simulink library "HDL_ieee_8021513"  (R2024a)
settings: Solver=FixedStepDiscrete  StartTime=0.0  StopTime=10.0  RelTol=1e-3
undefined symbols (not defined in the file): Add, axiWidth, CONST, fs, peakDetectorThreshold, peakDetectorWindow, QAM, Shift
libraries: hdlsllib x199, $bdroot x91, whdlutilities x34, whdledac x9, simulink x8, whdlmod x6, dspsigops x5, dsphdlfiltering2 x4, embreciprocals x3, dsphdlsigops2 x2, commhdlcrc x2, dspstat3 x2
(part 6 of 6)

== system HDL_ieee_8021513/full_tx/store_frame_in_ram/read_frame_from_ram/bits_selector ==
  rd_addr : Inport
  bits_per_subcarrier : Inport  Port=2
  Compare To Constant : hdlsllib/Logic and Bit Operations/Compare To Constant  relop=<=  const=CONST.preambleDataCarriers-1  OutDataTypeStr=boolean
  Compare To Constant1 : hdlsllib/Logic and Bit Operations/Compare To Constant  relop=<=  const=CONST.preambleDataCarriers + CONST.channelDataCarriers -1  OutDataTypeStr=boolean
  Compare To Constant2 : hdlsllib/Logic and Bit Operations/Compare To Constant  relop=<=  const=CONST.preambleDataCarriers + CONST.channelDataCarriers + CONST.headerDataCarriers-1  OutDataTypeStr=boolean
  Constant : Constant  OutDataTypeStr=fixdt(0,4,0)  SampleTime=-1
  Constant1 : Constant  OutDataTypeStr=fixdt(0,4,0)  SampleTime=-1
  Constant2 : Constant  Value=2  OutDataTypeStr=fixdt(0,4,0)  SampleTime=-1
  Delay{,1..5} (6 alike) : Delay  DelayLength=1  InitialCondition=0  UseCircularBuffer=on
  Multiport Switch : MultiPortSwitch  DataPortOrder=Zero-based contiguous  Inputs=4  zeroidx=on  SaturateOnIntegerOverflow=off  InputSameDT=off
  State Control : StateControl  StateControl=Synchronous
  one_hot_coder : Subsystem
  bits_per_subcarrier_out : Outport
  wires:
  Delay5/1 -> one_hot_coder/1(preamble)
  Delay4/1 -> one_hot_coder/2(channel)
  Delay3/1 -> one_hot_coder/3(header)
  Delay2/1 -> Delay1/1
  Delay1/1 -> Multiport Switch/5
  Compare To Constant1/1 -> Delay4/1
  one_hot_coder/1(bits_per_subcarrier_select) -> Delay/1
  Compare To Constant/1 -> Delay5/1
  Constant2/1 -> Multiport Switch/4
  Constant1/1 -> Multiport Switch/3
  Constant/1 -> Multiport Switch/2
  Compare To Constant2/1 -> Delay3/1
  rd_addr/1 -> Compare To Constant2/1, Compare To Constant/1, Compare To Constant1/1
  Multiport Switch/1 -> bits_per_subcarrier_out/1
  Delay/1 -> Multiport Switch/1
  bits_per_subcarrier/1 -> Delay2/1

== system HDL_ieee_8021513/full_tx/store_frame_in_ram/read_frame_from_ram/cp_len_creator ==
  rd_addr : Inport
  cp_len_in : Inport  Port=2
  Bits to Word : hdlsllib/Logic and Bit Operations/Bits to Word
  Compare To Constant : hdlsllib/Logic and Bit Operations/Compare To Constant  relop=<=  const=CONST.preambleDataCarriers-1  OutDataTypeStr=boolean
  Compare To Constant1 : hdlsllib/Logic and Bit Operations/Compare To Constant  relop=<=  const=CONST.preambleDataCarriers + CONST.channelDataCarriers -1  OutDataTypeStr=boolean
  Compare To Constant2 : hdlsllib/Logic and Bit Operations/Compare To Constant  relop=<=  const=CONST.preambleDataCarriers + CONST.channelDataCarriers + CONST.headerDataCarriers-1  OutDataTypeStr=boolean
  Constant : Constant  Value=CONST.preambleCyclicPrefixLen  OutDataTypeStr=uint8  SampleTime=-1
  Constant1 : Constant  Value=CONST.channelCyclicPrefixLen  OutDataTypeStr=uint8  SampleTime=-1
  Constant2 : Constant  Value=CONST.headerCyclicPrefixLen  OutDataTypeStr=uint8  SampleTime=-1
  Constant3 : Constant  Value=CONST.N/32  OutDataTypeStr=fixdt(0,4,0)  SampleTime=-1
  Data Type Conversion : DataTypeConversion  OutDataTypeStr=fixdt(0,1,0)  SaturateOnIntegerOverflow=off  RndMeth=Floor
  Delay{,1..5} (6 alike) : Delay  DelayLength=1  InitialCondition=0  UseCircularBuffer=on
  Delay6 : Delay  InitialCondition=0  UseCircularBuffer=on
  Multiport Switch : MultiPortSwitch  DataPortOrder=Zero-based contiguous  Inputs=4  zeroidx=on  OutDataTypeStr=uint8  SaturateOnIntegerOverflow=off
  Product : Product  OutDataTypeStr=uint8
  State Control : StateControl  StateControl=Synchronous
  one_hot_coder : Subsystem
  cp_len : Outport
  wires:
  Delay6/1 -> Product/2
  Delay5/1 -> one_hot_coder/1(preamble)
  Delay4/1 -> one_hot_coder/2(channel)
  Delay3/1 -> one_hot_coder/3(header)
  Delay2/1 -> Delay1/1
  rd_addr/1 -> Compare To Constant2/1, Compare To Constant/1, Compare To Constant1/1
  Compare To Constant/1 -> Delay5/1
  Compare To Constant1/1 -> Delay4/1
  Compare To Constant2/1 -> Delay3/1
  Constant/1 -> Multiport Switch/2
  Constant1/1 -> Multiport Switch/3
  Constant2/1 -> Multiport Switch/4
  Multiport Switch/1 -> cp_len/1
  one_hot_coder/1(cp_select) -> Delay/1
  Delay/1 -> Multiport Switch/1
  Constant3/1 -> Product/1
  cp_len_in/1 -> Data Type Conversion/1
  Product/1 -> Delay2/1
  Data Type Conversion/1 -> Bits to Word/1
  Bits to Word/1 -> Delay6/1
  Delay1/1 -> Multiport Switch/5

== system HDL_ieee_8021513/full_tx/store_frame_in_ram/read_frame_from_ram/init_selector ==
  rd_addr : Inport
  Compare To Constant : hdlsllib/Logic and Bit Operations/Compare To Constant  relop=<=  const=CONST.preambleDataCarriers-1  OutDataTypeStr=boolean
  Compare To Constant1 : hdlsllib/Logic and Bit Operations/Compare To Constant  relop=<=  const=CONST.preambleDataCarriers + CONST.channelDataCarriers -1  OutDataTypeStr=boolean
  Compare To Constant2 : hdlsllib/Logic and Bit Operations/Compare To Constant  relop=<=  const=CONST.preambleDataCarriers + CONST.channelDataCarriers + CONST.headerDataCarriers-1  OutDataTypeStr=boolean
  Constant : Constant  Value=CONST.preambleScramblerInit  OutDataTypeStr=boolean  SampleTime=-1
  Constant1 : Constant  Value=CONST.channelScramblerInit  OutDataTypeStr=boolean  SampleTime=-1
  Constant2 : Constant  Value=CONST.headerScramblerInit  OutDataTypeStr=boolean  SampleTime=-1
  Constant3 : Constant  Value=CONST.payloadScramblerInit  OutDataTypeStr=boolean  SampleTime=-1
  Delay{,1..3} (4 alike) : Delay  DelayLength=1  InitialCondition=0  UseCircularBuffer=on
  Multiport Switch : MultiPortSwitch  DataPortOrder=Zero-based contiguous  Inputs=4  zeroidx=on  SaturateOnIntegerOverflow=off  InputSameDT=off
  State Control : StateControl  StateControl=Synchronous
  one_hot_coder : Subsystem
  init : Outport
  wires:
  Delay3/1 -> one_hot_coder/1(preamble)
  Delay2/1 -> one_hot_coder/2(channel)
  Delay1/1 -> one_hot_coder/3(header)
  Compare To Constant1/1 -> Delay2/1
  one_hot_coder/1(cp_select) -> Delay/1
  Compare To Constant/1 -> Delay3/1
  Constant2/1 -> Multiport Switch/4
  Constant1/1 -> Multiport Switch/3
  Constant/1 -> Multiport Switch/2
  Compare To Constant2/1 -> Delay1/1
  rd_addr/1 -> Compare To Constant2/1, Compare To Constant/1, Compare To Constant1/1
  Multiport Switch/1 -> init/1
  Delay/1 -> Multiport Switch/1
  Constant3/1 -> Multiport Switch/5

== system HDL_ieee_8021513/full_tx/store_frame_in_ram/write_frame_to_ram/ram_formatting ==
  preamble_valid : Inport
  channel_valid : Inport  Port=2
  header_valid : Inport  Port=3
  payload_valid : Inport  Port=4
  preamble : Inport  Port=5
  channel : Inport  Port=6
  header : Inport  Port=7
  payload : Inport  Port=8
  Bit Concat{,1..2,6} (4 alike) : hdlsllib/Logic and Bit Operations/Bit Concat  numInputs=2
  Constant10 : Constant  Value=0  OutDataTypeStr=boolean  SampleTime=-1
  Constant11 : Constant  Value=0  OutDataTypeStr=boolean  SampleTime=-1
  Demux : Demux  Outputs=2
  Demux3 : Demux  Outputs=2
  Multiport Switch : MultiPortSwitch  DataPortOrder=Zero-based contiguous  Inputs=4  zeroidx=on  SaturateOnIntegerOverflow=off  InputSameDT=off
  State Control : StateControl  StateControl=Synchronous
  one_hot_coder : Subsystem
  Out1 : Outport
  wires:
  Demux3/2 -> Bit Concat6/2
  Demux3/1 -> Bit Concat6/1
  Demux/2 -> Bit Concat2/2
  Demux/1 -> Bit Concat2/1
  channel/1 -> Bit Concat1/2
  Constant11/1 -> Bit Concat1/1
  preamble/1 -> Bit Concat/2
  Constant10/1 -> Bit Concat/1
  header_valid/1 -> one_hot_coder/3(header_valid)
  Bit Concat1/1 -> Multiport Switch/3
  Bit Concat2/1 -> Multiport Switch/4
  header/1 -> Demux/1
  payload/1 -> Demux3/1
  one_hot_coder/1(data_select) -> Multiport Switch/1  "data_select"
  Bit Concat6/1 -> Multiport Switch/5
  channel_valid/1 -> one_hot_coder/2(channel_valid)
  preamble_valid/1 -> one_hot_coder/1(preamble_valid)
  Multiport Switch/1 -> Out1/1
  payload_valid/1 -> one_hot_coder/4(payload_valid)
  Bit Concat/1 -> Multiport Switch/2

== system HDL_ieee_8021513/full_tx/store_frame_in_ram/read_frame_from_ram/bits_selector/one_hot_coder ==
  preamble : Inport
  channel : Inport  Port=2
  header : Inport  Port=3
  Bit Concat : hdlsllib/Logic and Bit Operations/Bit Concat  numInputs=2
  Logical Operator : Logic  Operator=NOT  IconShape=distinctive  AllPortsSameDT=off  OutDataTypeStr=boolean
  Logical Operator1 : Logic  IconShape=distinctive  AllPortsSameDT=off  OutDataTypeStr=boolean
  Logical Operator2 : Logic  Operator=OR  IconShape=distinctive  AllPortsSameDT=off  OutDataTypeStr=boolean
  Logical Operator3 : Logic  Operator=NOT  IconShape=distinctive  AllPortsSameDT=off  OutDataTypeStr=boolean
  Logical Operator4 : Logic  Operator=NOT  IconShape=distinctive  AllPortsSameDT=off  OutDataTypeStr=boolean
  State Control : StateControl  StateControl=Synchronous
  bits_per_subcarrier_select : Outport
  wires:
  Bit Concat/1 -> bits_per_subcarrier_select/1
  channel/1 -> Logical Operator1/2, Logical Operator/1
  preamble/1 -> Logical Operator3/1
  Logical Operator3/1 -> Logical Operator1/1
  header/1 -> Logical Operator4/1
  Logical Operator1/1 -> Logical Operator2/1
  Logical Operator4/1 -> Logical Operator2/2
  Logical Operator/1 -> Bit Concat/1
  Logical Operator2/1 -> Bit Concat/2

== system HDL_ieee_8021513/full_tx/store_frame_in_ram/read_frame_from_ram/cp_len_creator/one_hot_coder ==
  preamble : Inport
  channel : Inport  Port=2
  header : Inport  Port=3
  Bit Concat : hdlsllib/Logic and Bit Operations/Bit Concat  numInputs=2
  Logical Operator : Logic  Operator=NOT  IconShape=distinctive  AllPortsSameDT=off  OutDataTypeStr=boolean
  Logical Operator1 : Logic  IconShape=distinctive  AllPortsSameDT=off  OutDataTypeStr=boolean
  Logical Operator2 : Logic  Operator=OR  IconShape=distinctive  AllPortsSameDT=off  OutDataTypeStr=boolean
  Logical Operator3 : Logic  Operator=NOT  IconShape=distinctive  AllPortsSameDT=off  OutDataTypeStr=boolean
  Logical Operator4 : Logic  Operator=NOT  IconShape=distinctive  AllPortsSameDT=off  OutDataTypeStr=boolean
  State Control : StateControl  StateControl=Synchronous
  cp_select : Outport
  wires:
  channel/1 -> Logical Operator1/2, Logical Operator/1
  Logical Operator/1 -> Bit Concat/1
  preamble/1 -> Logical Operator3/1
  Logical Operator3/1 -> Logical Operator1/1
  header/1 -> Logical Operator4/1
  Logical Operator1/1 -> Logical Operator2/1
  Logical Operator2/1 -> Bit Concat/2
  Logical Operator4/1 -> Logical Operator2/2
  Bit Concat/1 -> cp_select/1

== system HDL_ieee_8021513/full_tx/store_frame_in_ram/read_frame_from_ram/init_selector/one_hot_coder ==
  preamble : Inport
  channel : Inport  Port=2
  header : Inport  Port=3
  Bit Concat : hdlsllib/Logic and Bit Operations/Bit Concat  numInputs=2
  Logical Operator : Logic  Operator=NOT  IconShape=distinctive  AllPortsSameDT=off  OutDataTypeStr=boolean
  Logical Operator1 : Logic  IconShape=distinctive  AllPortsSameDT=off  OutDataTypeStr=boolean
  Logical Operator2 : Logic  Operator=OR  IconShape=distinctive  AllPortsSameDT=off  OutDataTypeStr=boolean
  Logical Operator3 : Logic  Operator=NOT  IconShape=distinctive  AllPortsSameDT=off  OutDataTypeStr=boolean
  Logical Operator4 : Logic  Operator=NOT  IconShape=distinctive  AllPortsSameDT=off  OutDataTypeStr=boolean
  State Control : StateControl  StateControl=Synchronous
  cp_select : Outport
  wires:
  Bit Concat/1 -> cp_select/1
  channel/1 -> Logical Operator1/2, Logical Operator/1
  preamble/1 -> Logical Operator3/1
  Logical Operator3/1 -> Logical Operator1/1
  header/1 -> Logical Operator4/1
  Logical Operator1/1 -> Logical Operator2/1
  Logical Operator4/1 -> Logical Operator2/2
  Logical Operator/1 -> Bit Concat/1
  Logical Operator2/1 -> Bit Concat/2

== system HDL_ieee_8021513/full_tx/store_frame_in_ram/write_frame_to_ram/ram_formatting/one_hot_coder ==
  preamble_valid : Inport
  channel_valid : Inport  Port=2
  header_valid : Inport  Port=3
  payload_valid : Inport  Port=4
  Bit Concat : hdlsllib/Logic and Bit Operations/Bit Concat  numInputs=2
  Logical Operator : Logic  Operator=OR  IconShape=distinctive  AllPortsSameDT=off  OutDataTypeStr=boolean
  Logical Operator1 : Logic  Operator=OR  IconShape=distinctive  AllPortsSameDT=off  OutDataTypeStr=boolean
  State Control : StateControl  StateControl=Synchronous
  Terminator : Terminator
  data_select : Outport
  wires:
  Bit Concat/1 -> data_select/1
  header_valid/1 -> Logical Operator/1
  channel_valid/1 -> Logical Operator1/2
  payload_valid/1 -> Logical Operator/2, Logical Operator1/1
  preamble_valid/1 -> Terminator/1
  Logical Operator1/1 -> Bit Concat/2
  Logical Operator/1 -> Bit Concat/1
